simulink model "LoadAnalyser"  (R2015b)
settings: Solver=FixedStepAuto  StartTime=0.0  StopTime=10  FixedStep=0.02  RelTol=1e-3
InitFcn:
  | ControlInit;
StopFcn:
  | PhasPlot;
values from neighbouring files (symbols this model uses):
  Rad2Deg = 180/pi    (= 57.2956455309)    [ControlInit.m]
undefined symbols (not defined in the file or in its folder): Imag, Real
libraries: powerlib x9, simulink x2
settings Model: Creator=Emilio  LastModifiedBy=Emilio

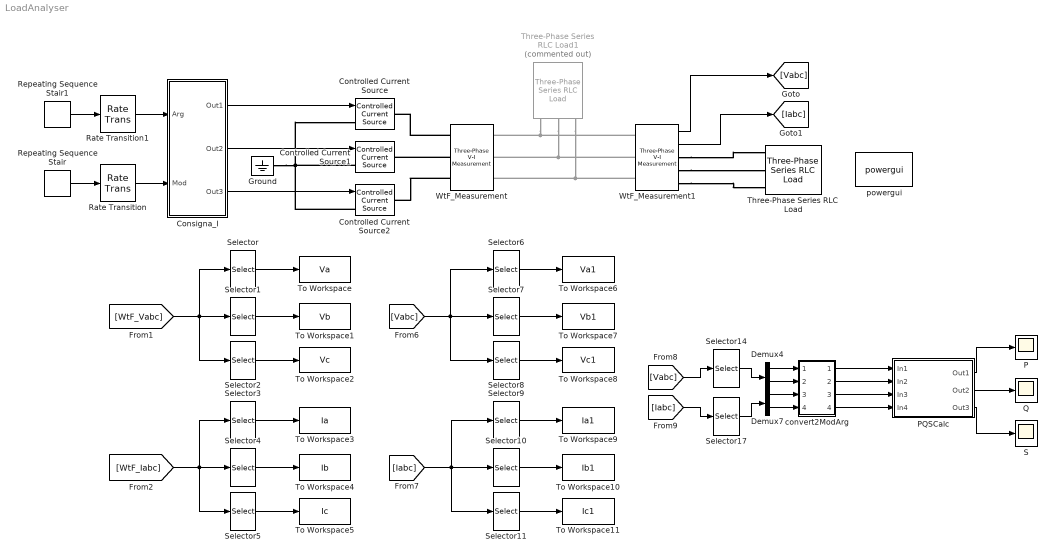
== system LoadAnalyser ==
  Consigna_I : Subsystem
  Controlled Current Source : powerlib/Electrical Sources/Controlled Current Source  Initialize=off  Source_Type=AC  Amplitude=0  Phase=0  Frequency=0  Measurements=None
  Controlled Current Source1 : powerlib/Electrical Sources/Controlled Current Source  Initialize=off  Source_Type=AC  Amplitude=0  Phase=0  Frequency=0  Measurements=None
  Controlled Current Source2 : powerlib/Electrical Sources/Controlled Current Source  Initialize=off  Source_Type=AC  Amplitude=0  Phase=0  Frequency=0  Measurements=None
  Demux4 : Demux  Outputs=2
  Demux7 : Demux  Outputs=2
  Ground : powerlib/Elements/Ground  LConnTagsString=a
  P : Scope
  PQSCalc : Subsystem
  Q : Scope
  Rate Transition : RateTransition  X0=100
  Rate Transition1 : RateTransition
  Repeating Sequence Stair : simulink/Sources/Repeating Sequence Stair  OutValues=[100 120 95 105].'  tsamp=2  OutMin=[]  OutMax=[]  OutDataTypeStr=double  OutputDataTypeScalingMode=double  OutDataType=fixdt(0,8)  ConRadixGroup=Best Precision: Vector-wise  OutScaling=2^-12
  Repeating Sequence Stair1 : simulink/Sources/Repeating Sequence Stair  OutValues=[0 30 60 90 70 45 20].'  tsamp=0.8  OutMin=[]  OutMax=[]  OutDataTypeStr=double  OutputDataTypeScalingMode=double  OutDataType=fixdt(0,8)  ConRadixGroup=Best Precision: Vector-wise  OutScaling=2^-12
  S : Scope
  Selector{,3,6,9,14,17} (6 alike) : Selector  InputPortWidth=6  IndexOptions=Index vector (dialog)  Indices=[1 4]  OutputSizes=1
  Selector{1,4,7,10} (4 alike) : Selector  InputPortWidth=6  IndexOptions=Index vector (dialog)  Indices=[2 5]  OutputSizes=1
  Selector{2,5,8,11} (4 alike) : Selector  InputPortWidth=6  IndexOptions=Index vector (dialog)  Indices=[3 6]  OutputSizes=1
  Three-Phase Series RLC Load : powerlib/Elements/Three-Phase Series RLC Load  LConnTagsString=A|B|C  Configuration=Y (grounded)  NominalVoltage=10  Vabc=[1e3 1e3 1e3]  Vabcp=[1e3 1e3 1e3]  NominalFrequency=50  UnbalancedPower=off  ActivePower=100  InductivePower=0  CapacitivePower=100  Pabc=[10e3 9e3 11e3]  QLabc=[100 90 110]  QCabc=[100 90 110]  Pabcp=[10e3 9e3 11e3]  QLabcp=[100 90 110]  QCabcp=[100 90 110]  Measurements=None  LoadType=constant Z
  Three-Phase Series RLC Load1 : powerlib/Elements/Three-Phase Series RLC Load  Commented=on  LConnTagsString=A|B|C  Configuration=Y (grounded)  NominalVoltage=10  Vabc=[1e3 1e3 1e3]  Vabcp=[1e3 1e3 1e3]  NominalFrequency=50  UnbalancedPower=off  ActivePower=50  InductivePower=0  CapacitivePower=0  Pabc=[10e3 9e3 11e3]  QLabc=[100 90 110]  QCabc=[100 90 110]  Pabcp=[10e3 9e3 11e3]  QLabcp=[100 90 110]  QCabcp=[100 90 110]  Measurements=None  LoadType=constant Z
  To Workspace : ToWorkspace  VariableName=Va  SampleTime=-1
  To Workspace1 : ToWorkspace  VariableName=Vb  SampleTime=-1
  To Workspace10 : ToWorkspace  VariableName=Ib1  SampleTime=-1
  To Workspace11 : ToWorkspace  VariableName=Ic1  SampleTime=-1
  To Workspace2 : ToWorkspace  VariableName=Vc  SampleTime=-1
  To Workspace3 : ToWorkspace  VariableName=Ia  SampleTime=-1
  To Workspace4 : ToWorkspace  VariableName=Ib  SampleTime=-1
  To Workspace5 : ToWorkspace  VariableName=Ic  SampleTime=-1
  To Workspace6 : ToWorkspace  VariableName=Va1  SampleTime=-1
  To Workspace7 : ToWorkspace  VariableName=Vb1  SampleTime=-1
  To Workspace8 : ToWorkspace  VariableName=Vc1  SampleTime=-1
  To Workspace9 : ToWorkspace  VariableName=Ia1  SampleTime=-1
  WtF_Measurement : powerlib/Measurements/Three-Phase V-I Measurement  VoltageMeasurement=phase-to-ground  SetLabelV=on  LabelV=WtF_Vabc  Vpu=off  VpuLL=off  CurrentMeasurement=yes  SetLabelI=on  LabelI=WtF_Iabc  Ipu=off  Pbase=100e6  Vbase=500e3  OutputType=Real-Imag  PhasorSimulation=on  PSBequivalent=0
  WtF_Measurement1 : powerlib/Measurements/Three-Phase V-I Measurement  VoltageMeasurement=phase-to-ground  SetLabelV=off  LabelV=WtF_Vabc  Vpu=off  VpuLL=off  CurrentMeasurement=yes  SetLabelI=off  LabelI=WtF_Iabc  Ipu=off  Pbase=100e6  Vbase=500e3  OutputType=Real-Imag  PhasorSimulation=on  PSBequivalent=0
  convert2ModArg : Subsystem
  powergui : powerlib/powergui  Priority=1  SimulationMode=Phasor  SolverType=Tustin/Backward Euler (TBE)  SampleTime=50e-6  frequency=Fnom  SPID=off  DisableSnubberDevices=off  DisableRonSwitches=off  DisableVfSwitches=off  SwTol=0  DisplayEquations=off  Interpol=off  ExternalGateDelay=off  methode=off  Ts=10  FunctionMessages=off  echomessages=off  HookPort=off  EnableUseOfTLC=off  x0status=blocks  frequencyindice=50  Pbase=100e6  ErrMax=1e-4  Iterations=50  UnitsV=V  UnitsW=W  buscounter=0  RestoreLinks=warning  ResistiveCurrentMeasurement=off  Frange=[0:2:500]  Ylog=off  Xlog=on  ShowGrid=off  save=off  variable=ZData  structure=0  ZoomFFT=off  StartTime=0.0  cycles=1  DisplayStyle=1  fundamental=60  FreqAxis=off  MaxFrequency=1000  frequencyindicesteady=1  RmsSteady=1  display=off
  wires:
  Consigna_I/1(Out1) -> Controlled Current Source/1
  Consigna_I/2(Out2) -> Controlled Current Source1/1
  Consigna_I/3(Out3) -> Controlled Current Source2/1
  [WtF_Vabc] -> Selector/1, Selector2/1, Selector1/1
  Selector/1 -> To Workspace/1
  Selector1/1 -> To Workspace1/1
  Selector2/1 -> To Workspace2/1
  [WtF_Iabc] -> Selector4/1, Selector5/1, Selector3/1
  Selector3/1 -> To Workspace3/1
  Selector4/1 -> To Workspace4/1
  Selector5/1 -> To Workspace5/1
  Selector6/1 -> To Workspace6/1
  Selector7/1 -> To Workspace7/1
  Selector8/1 -> To Workspace8/1
  Selector9/1 -> To Workspace9/1
  Selector10/1 -> To Workspace10/1
  Selector11/1 -> To Workspace11/1
  WtF_Measurement1/2 -> [Iabc]
  WtF_Measurement1/1 -> [Vabc]
  [Vabc] -> Selector8/1, Selector7/1, Selector6/1
  [Iabc] -> Selector11/1, Selector9/1, Selector10/1
  [Vabc] -> Selector14/1
  [Iabc] -> Selector17/1
  Selector14/1 -> Demux4/1
  Selector17/1 -> Demux7/1
  Demux4/1 -> convert2ModArg/1(In1)
  Demux4/2 -> convert2ModArg/2(In2)
  Demux7/1 -> convert2ModArg/3(In3)
  Demux7/2 -> convert2ModArg/4(In4)
  convert2ModArg/1(Out1) -> PQSCalc/1(In1)
  convert2ModArg/2(Out2) -> PQSCalc/2(In2)
  convert2ModArg/3(Out3) -> PQSCalc/3(In3)
  convert2ModArg/4(Out4) -> PQSCalc/4(In4)
  PQSCalc/1(Out1) -> P/1
  PQSCalc/2(Out2) -> Q/1
  PQSCalc/3(Out3) -> S/1
  Repeating Sequence Stair/1 -> Rate Transition/1
  Repeating Sequence Stair1/1 -> Rate Transition1/1
  Rate Transition1/1 -> Consigna_I/1(Arg)
  Rate Transition/1 -> Consigna_I/2(Mod)
  connections:
  WtF_Measurement/LConn2 -- Controlled Current Source1/RConn1
  Three-Phase Series RLC Load1/LConn3 -- WtF_Measurement1/LConn3 -- WtF_Measurement/RConn3
  Three-Phase Series RLC Load1/LConn2 -- WtF_Measurement1/LConn2 -- WtF_Measurement/RConn2
  WtF_Measurement/LConn3 -- Controlled Current Source2/RConn1
  WtF_Measurement/LConn1 -- Controlled Current Source/RConn1
  Three-Phase Series RLC Load1/LConn1 -- WtF_Measurement1/LConn1 -- WtF_Measurement/RConn1
  Controlled Current Source2/LConn1 -- Ground/LConn1 -- Controlled Current Source/LConn1 -- Controlled Current Source1/LConn1
  WtF_Measurement1/RConn2 -- Three-Phase Series RLC Load/LConn2
  WtF_Measurement1/RConn3 -- Three-Phase Series RLC Load/LConn3
  WtF_Measurement1/RConn1 -- Three-Phase Series RLC Load/LConn1

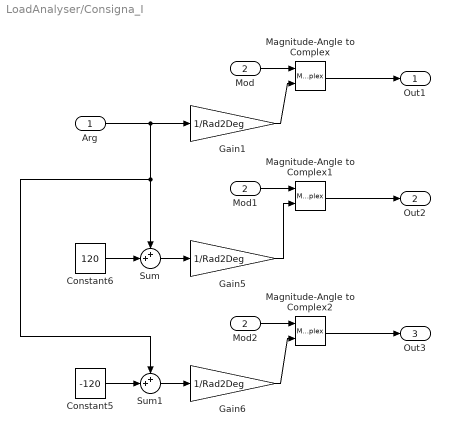
== system LoadAnalyser/Consigna_I ==
  Arg : Inport
  Mod : Inport  Port=2
  Constant5 : Constant  Value=-120
  Constant6 : Constant  Value=120
  Gain1 : Gain  Gain=1/Rad2Deg
  Gain5 : Gain  Gain=1/Rad2Deg
  Gain6 : Gain  Gain=1/Rad2Deg
  Magnitude-Angle to Complex : MagnitudeAngleToComplex
  Magnitude-Angle to Complex1 : MagnitudeAngleToComplex
  Magnitude-Angle to Complex2 : MagnitudeAngleToComplex
  Mod1 : InportShadow  Port=2
  Mod2 : InportShadow  Port=2
  Sum : Sum  Inputs=++|
  Sum1 : Sum  Inputs=++|
  Out1 : Outport
  Out2 : Outport  Port=2
  Out3 : Outport  Port=3
  wires:
  Gain1/1 -> Magnitude-Angle to Complex/2
  Constant6/1 -> Sum/2
  Sum/1 -> Gain5/1
  Constant5/1 -> Sum1/2
  Sum1/1 -> Gain6/1
  Arg/1 -> Sum1/1, Sum/1, Gain1/1
  Mod/1 -> Magnitude-Angle to Complex/1
  Mod1/1 -> Magnitude-Angle to Complex1/1
  Mod2/1 -> Magnitude-Angle to Complex2/1
  Gain6/1 -> Magnitude-Angle to Complex2/2
  Gain5/1 -> Magnitude-Angle to Complex1/2
  Magnitude-Angle to Complex2/1 -> Out3/1
  Magnitude-Angle to Complex1/1 -> Out2/1
  Magnitude-Angle to Complex/1 -> Out1/1

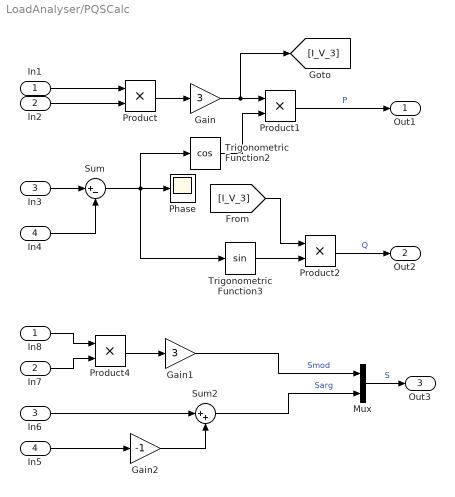
== system LoadAnalyser/PQSCalc ==
  In1 : Inport
  In2 : Inport  Port=2
  In3 : Inport  Port=3
  In4 : Inport  Port=4
  Gain : Gain  Gain=3
  Gain1 : Gain  Gain=3
  Gain2 : Gain  Gain=-1
  In5 : InportShadow  Port=4
  In6 : InportShadow  Port=3
  In7 : InportShadow  Port=2
  In8 : InportShadow
  Mux : Mux  Inputs=2
  Phase : Scope
  Product{,1..2,4} (4 alike) : Product
  Sum : Sum  Inputs=|+-
  Sum2 : Sum  Inputs=|++
  Trigonometric Function2 : Trigonometry  Operator=cos
  Trigonometric Function3 : Trigonometry
  Out1 : Outport
  Out2 : Outport  Port=2
  Out3 : Outport  Port=3
  wires:
  Product/1 -> Gain/1
  Gain/1 -> [I_V_3], Product1/1
  Trigonometric Function2/1 -> Product1/2
  Product1/1 -> Out1/1  "P"
  Sum/1 -> Phase/1, Trigonometric Function3/1, Trigonometric Function2/1
  Product2/1 -> Out2/1  "Q"
  Trigonometric Function3/1 -> Product2/2
  In3/1 -> Sum/1
  In1/1 -> Product/1
  In2/1 -> Product/2
  In4/1 -> Sum/2
  [I_V_3] -> Product2/1
  In8/1 -> Product4/1
  Product4/1 -> Gain1/1
  In7/1 -> Product4/2
  Gain1/1 -> Mux/1  "Smod"
  In5/1 -> Gain2/1
  In6/1 -> Sum2/1
  Gain2/1 -> Sum2/2
  Sum2/1 -> Mux/2  "Sarg"
  Mux/1 -> Out3/1  "S"

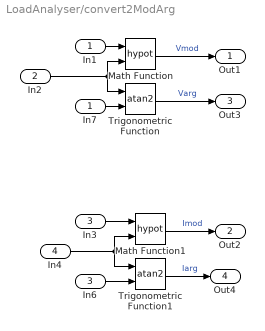
== system LoadAnalyser/convert2ModArg ==
  In1 : Inport
  In2 : Inport  Port=2
  In3 : Inport  Port=3
  In4 : Inport  Port=4
  In6 : InportShadow  Port=3
  In7 : InportShadow
  Math Function : Math  Operator=hypot  SaturateOnIntegerOverflow=on
  Math Function1 : Math  Operator=hypot  SaturateOnIntegerOverflow=on
  Trigonometric Function : Trigonometry  Operator=atan2
  Trigonometric Function1 : Trigonometry  Operator=atan2
  Out1 : Outport
  Out2 : Outport  Port=2
  Out3 : Outport  Port=3
  Out4 : Outport  Port=4
  wires:
  In2/1 -> Math Function/2, Trigonometric Function/1
  In1/1 -> Math Function/1
  Math Function1/1 -> Out2/1  "Imod"
  Trigonometric Function1/1 -> Out4/1  "Iarg"
  Trigonometric Function/1 -> Out3/1  "Varg"
  Math Function/1 -> Out1/1  "Vmod"
  In4/1 -> Math Function1/2, Trigonometric Function1/1
  In3/1 -> Math Function1/1
  In6/1 -> Trigonometric Function1/2
  In7/1 -> Trigonometric Function/2
